simulink model "Baxter_Dyn_PID_2020"  (R2020a)
settings: Solver=FixedStepDiscrete  StartTime=0.0  StopTime=30  FixedStep=0.02  RelTol=1e-3
InitFcn:
  | initGoals
StopFcn:
  | plotSimBaxter
model workspace (MAT data in the model file):
  SL_ROS_VariableLengthArrays_MaxSizes.CommonInfo.ArrayTruncateAction = 'EmitWarning'
  SL_ROS_VariableLengthArrays_MaxSizes.MsgTypeMap = containers.Map
  SL_ROS_VariableLengthArrays_MaxSizes.MsgTypeMap.serialization.keys = {'baxter_core_msgs/JointCommand', 'sensor_msgs/JointState'}
  SL_ROS_VariableLengthArrays_MaxSizes.MsgTypeMap.serialization.values{1}(1).PropertyName = 'Command'
  SL_ROS_VariableLengthArrays_MaxSizes.MsgTypeMap.serialization.values{1}(1).DataType = 'double'
  SL_ROS_VariableLengthArrays_MaxSizes.MsgTypeMap.serialization.values{1}(1).MaxLength = 128
  SL_ROS_VariableLengthArrays_MaxSizes.MsgTypeMap.serialization.values{1}(2).PropertyName = 'Names'
  SL_ROS_VariableLengthArrays_MaxSizes.MsgTypeMap.serialization.values{1}(2).DataType = 'std_msgs/String'
  SL_ROS_VariableLengthArrays_MaxSizes.MsgTypeMap.serialization.values{1}(2).MaxLength = 19
  SL_ROS_VariableLengthArrays_MaxSizes.MsgTypeMap.serialization.values{2}(1).PropertyName = 'Effort'
  SL_ROS_VariableLengthArrays_MaxSizes.MsgTypeMap.serialization.values{2}(1).DataType = 'double'
  SL_ROS_VariableLengthArrays_MaxSizes.MsgTypeMap.serialization.values{2}(1).MaxLength = 128
  SL_ROS_VariableLengthArrays_MaxSizes.MsgTypeMap.serialization.values{2}(2).PropertyName = 'Name'
  SL_ROS_VariableLengthArrays_MaxSizes.MsgTypeMap.serialization.values{2}(2).DataType = 'std_msgs/String'
  SL_ROS_VariableLengthArrays_MaxSizes.MsgTypeMap.serialization.values{2}(2).MaxLength = 19
  SL_ROS_VariableLengthArrays_MaxSizes.MsgTypeMap.serialization.values{2}(3).PropertyName = 'Position'
  SL_ROS_VariableLengthArrays_MaxSizes.MsgTypeMap.serialization.values{2}(3).DataType = 'double'
  SL_ROS_VariableLengthArrays_MaxSizes.MsgTypeMap.serialization.values{2}(3).MaxLength = 19
  SL_ROS_VariableLengthArrays_MaxSizes.MsgTypeMap.serialization.values{2}(4).PropertyName = 'Velocity'
  SL_ROS_VariableLengthArrays_MaxSizes.MsgTypeMap.serialization.values{2}(4).DataType = 'double'
  SL_ROS_VariableLengthArrays_MaxSizes.MsgTypeMap.serialization.values{2}(4).MaxLength = 19
  SL_ROS_VariableLengthArrays_MaxSizes.MsgTypeMap.serialization.uniformity = 0
  SL_ROS_VariableLengthArrays_MaxSizes.MsgTypeMap.serialization.keyType = 'char'
  SL_ROS_VariableLengthArrays_MaxSizes.MsgTypeMap.serialization.valueType = 'any'
values from neighbouring files (symbols this model uses):
  Kp = [  1,0,0,0,0,0,0;         0,1,0,0,0,0,0;         0,0,1,0,0,0,0;         0,0,0,1,0,0,0;         0,0,0,0,1,0,0;         0,0,0,0,0,1,0;         0,0,0,0,0,0,1]    [initGoals.m]
  Kv = [  0,0,0,0,0,0,0;         0,0,0,0,0,0,0;         0,0,0,0,0,0,0;         0,0,0,0,0,0,0;         0,0,0,0,0,0,0;         0,0,0,0,0,0,0;         0,0,0,0,0,0,0]    [initGoals.m]
libraries: simulink x7, lab3lib x4
settings Model: Creator=jcollial  LastModifiedBy=spkee
settings OptimizationCC: EnhancedBackFolding=on  PassReuseOutputArgsAs=Individual arguments  ZeroExternalMemoryAtStartup=off  ZeroInternalMemoryAtStartup=off  MaxStackSize=64  OptimizeBlockOrder=speed  DifferentSizesBufferReuse=on  OptimizationCustomize=off  EfficientTunableParamExpr=on
settings DebuggingCC: ParameterTunabilityLossMsg=error
settings HardwareCC: ProdBitPerPointer=32  ProdBitPerSizeT=32  ProdBitPerPtrDiffT=32  ProdLargestAtomicFloat=None  ProdIntDivRoundTo=Undefined  ProdEndianess=Unspecified  ProdWordSize=32  ProdHWDeviceType=Generic->Unspecified (assume 32-bit Generic)  UseEmbeddedCoderFeatures=off
settings SFSimCC: MATLABDynamicMemAlloc=off
settings RTWCC: SystemTargetFile=ert.tlc  HardwareBoard=Robot Operating System (ROS)  TemplateMakefile=ert_default_tmf  Toolchain=Catkin  TargetLang=C++
settings CodeAppCC: ForceParamTrailComments=on  IgnoreCustomStorageClasses=off  OperatorAnnotations=on  SimulinkDataObjDesc=on  SFDataObjDesc=on  InsertBlockDesc=on
settings ERTTargetCC: SupportNonInlinedSFcns=on

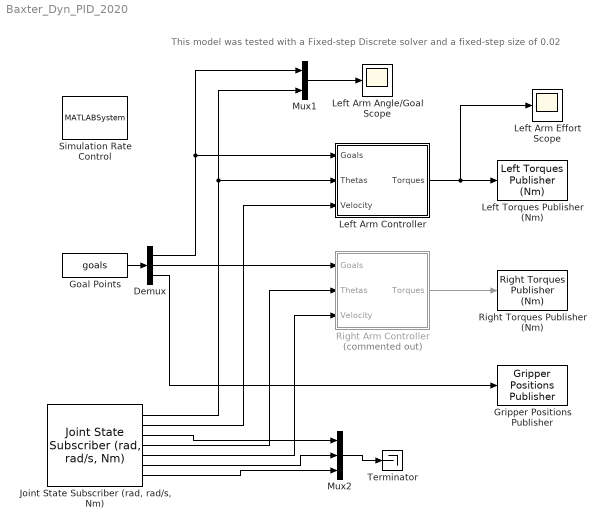
== system Baxter_Dyn_PID_2020 ==
  note: This model was tested with a Fixed-step Discrete solver and a fixed-step size of 0.02
  Demux : Demux  Outputs=3
  Goal Points : FromWorkspace  VariableName=goals  Interpolate=off  OutputAfterFinalValue=Holding final value
  Gripper Positions Publisher : lab3lib/Gripper Positions Publisher
      link override Publish: topic=/robot/end_effector/left_gripper/command  messageType=baxter_core_msgs/EndEffectorCommand
      settings: SourceProductName=Baxter
  "Joint State Subscriber (rad, rad/s, Nm)" : lab3lib/Joint State Subscriber (rad, rad//s, Nm)
      settings: SourceProductName=Baxter
  Left Arm Angle/Goal Scope : Scope
  Left Arm Controller : Subsystem
  Left Arm Effort Scope : Scope
  Left Torques Publisher (Nm) : lab3lib/Left Torques Publisher (Nm)
      settings: SourceProductName=Baxter
  Mux1 : Mux  Inputs=2
  Mux2 : Mux  Inputs=3
  Right Arm Controller : Subsystem  Commented=on
  Right Torques Publisher (Nm) : lab3lib/Right Torques Publisher (Nm)
      settings: SourceProductName=Baxter
  Simulation Rate Control : MATLABSystem  System=ExampleHelperSimulationRateControl  SampleTime=0.02
      mask Type: ExampleHelperSimulationRateControl
      mask Display: disp('Rate Control');
  Terminator : Terminator
  wires:
  Demux/1 -> Left Arm Controller/1(Goals), Mux1/1
  "Joint State Subscriber (rad, rad/s, Nm)"/1 -> Left Arm Controller/2(Thetas), Mux1/2
  Mux1/1 -> Left Arm Angle/Goal Scope/1
  Mux2/1 -> Terminator/1
  Goal Points/1 -> Demux/1
  Demux/3 -> Gripper Positions Publisher/1
  Left Arm Controller/1(Torques) -> Left Torques Publisher (Nm)/1, Left Arm Effort Scope/1
  "Joint State Subscriber (rad, rad/s, Nm)"/2 -> Left Arm Controller/3(Velocity)
  Demux/2 -> Right Arm Controller/1(Goals)
  Right Arm Controller/1(Torques) -> Right Torques Publisher (Nm)/1
  "Joint State Subscriber (rad, rad/s, Nm)"/4 -> Right Arm Controller/2(Thetas)
  "Joint State Subscriber (rad, rad/s, Nm)"/5 -> Right Arm Controller/3(Velocity)
  "Joint State Subscriber (rad, rad/s, Nm)"/3 -> Mux2/1
  "Joint State Subscriber (rad, rad/s, Nm)"/6 -> Mux2/2
  "Joint State Subscriber (rad, rad/s, Nm)"/7 -> Mux2/3

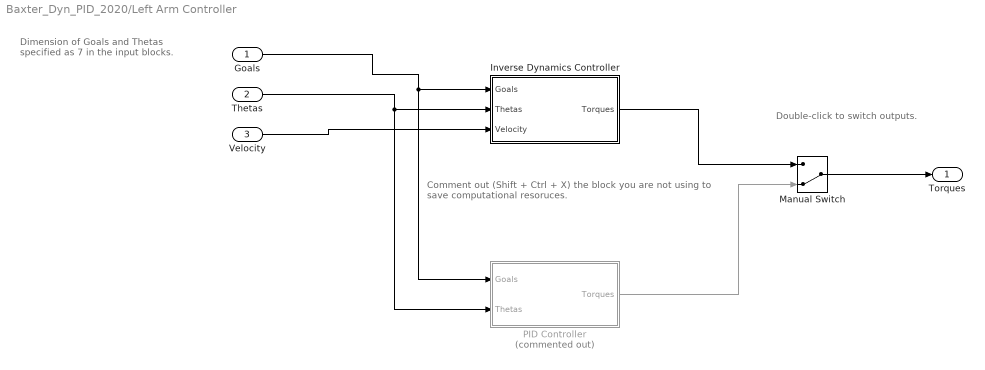
== system Baxter_Dyn_PID_2020/Left Arm Controller ==
  note: Dimension of Goals and Thetas
      | specified as 7 in the input blocks.
  note: Comment out (Shift + Ctrl + X) the block you are not using
      | to save computational resoruces.
  note: Double-click to switch outputs.
  Goals : Inport  PortDimensions=7
  Thetas : Inport  Port=2  PortDimensions=7
  Velocity : Inport  Port=3  PortDimensions=7
  Inverse Dynamics Controller : Subsystem
  Manual Switch : ManualSwitch  CurrentSetting=0
  PID Controller : Subsystem  Commented=on
  Torques : Outport
  wires:
  Goals/1 -> PID Controller/1(Goals), Inverse Dynamics Controller/1(Goals)
  Thetas/1 -> PID Controller/2(Thetas), Inverse Dynamics Controller/2(Thetas)
  Velocity/1 -> Inverse Dynamics Controller/3(Velocity)
  Manual Switch/1 -> Torques/1
  Inverse Dynamics Controller/1(Torques) -> Manual Switch/1
  PID Controller/1(Torques) -> Manual Switch/2

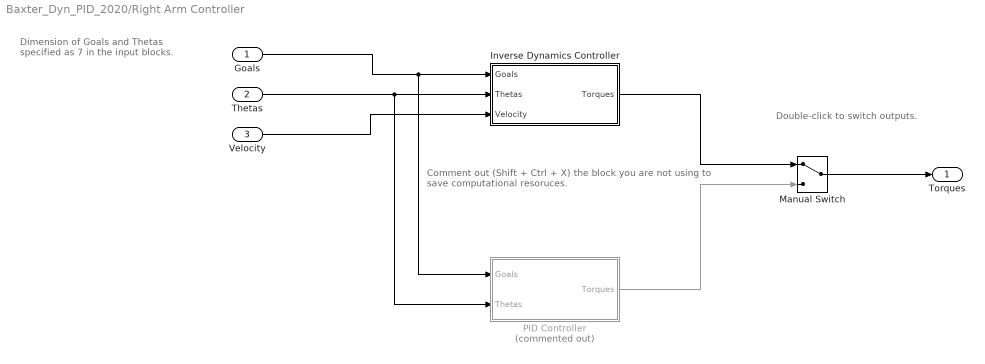
== system Baxter_Dyn_PID_2020/Right Arm Controller ==
  note: Double-click to switch outputs.
  note: Comment out (Shift + Ctrl + X) the block you are not using
      | to save computational resoruces.
  note: Dimension of Goals and Thetas
      | specified as 7 in the input blocks.
  Goals : Inport  PortDimensions=7
  Thetas : Inport  Port=2  PortDimensions=7
  Velocity : Inport  Port=3  PortDimensions=7
  Inverse Dynamics Controller : Subsystem
  Manual Switch : ManualSwitch
  PID Controller : Subsystem  Commented=on
  Torques : Outport
  wires:
  PID Controller/1(Torques) -> Manual Switch/2
  Thetas/1 -> PID Controller/2(Thetas), Inverse Dynamics Controller/2(Thetas)
  Inverse Dynamics Controller/1(Torques) -> Manual Switch/1
  Velocity/1 -> Inverse Dynamics Controller/3(Velocity)
  Goals/1 -> PID Controller/1(Goals), Inverse Dynamics Controller/1(Goals)
  Manual Switch/1 -> Torques/1

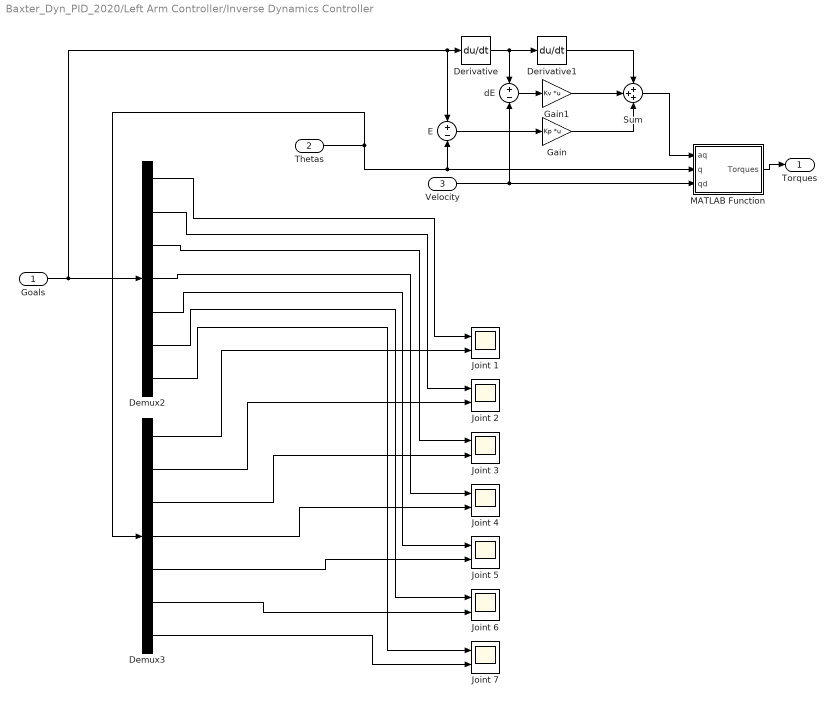
== system Baxter_Dyn_PID_2020/Left Arm Controller/Inverse Dynamics Controller ==
  Goals : Inport  PortDimensions=7
  Thetas : Inport  Port=2  PortDimensions=7
  Velocity : Inport  Port=3  PortDimensions=7
  Demux2 : Demux  Outputs=7
  Demux3 : Demux  Outputs=7
  Derivative : Derivative
  Derivative1 : Derivative
  E : Sum  Inputs=+|-
  Gain : Gain  Gain=Kp  Multiplication=Matrix(K*u)
  Gain1 : Gain  Gain=Kv  Multiplication=Matrix(K*u)
  Joint {1..7} (7 alike) : Scope  NumInputPorts=2
  MATLAB Function : MATLAB Function  TreatAsAtomicUnit=on
  Sum : Sum  Inputs=+++
  dE : Sum  Inputs=+|-
  Torques : Outport
  wires:
  MATLAB Function/1(Torques) -> Torques/1
  Demux3/3 -> Joint 3/2
  Gain/1 -> Sum/3
  Derivative1/1 -> Sum/1
  Thetas/1 -> Demux3/1, E/2, MATLAB Function/2(q)
  Derivative/1 -> Derivative1/1, dE/1
  Demux2/4 -> Joint 4/1
  Demux3/4 -> Joint 4/2
  Goals/1 -> Derivative/1, E/1, Demux2/1
  Velocity/1 -> MATLAB Function/3(qd), dE/2
  Demux3/5 -> Joint 5/2
  Demux2/1 -> Joint 1/1
  Gain1/1 -> Sum/2
  Demux3/1 -> Joint 1/2
  Demux3/7 -> Joint 7/2
  Demux3/6 -> Joint 6/2
  Demux2/3 -> Joint 3/1
  Demux2/2 -> Joint 2/1
  Demux2/6 -> Joint 6/1
  E/1 -> Gain/1
  Demux2/7 -> Joint 7/1
  Demux3/2 -> Joint 2/2
  Demux2/5 -> Joint 5/1
  dE/1 -> Gain1/1
  Sum/1 -> MATLAB Function/1(aq)

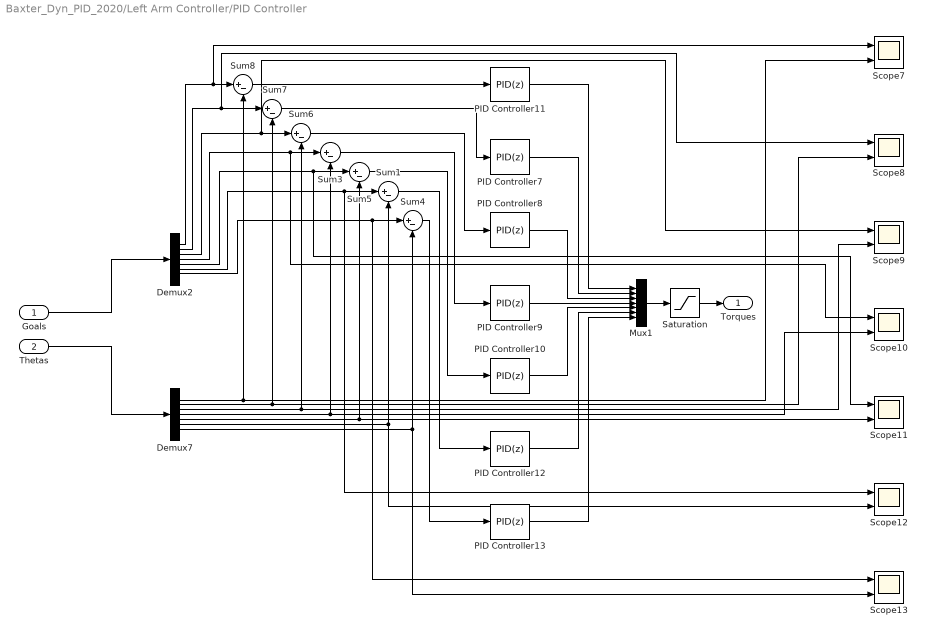
== system Baxter_Dyn_PID_2020/Left Arm Controller/PID Controller ==
  Goals : Inport  PortDimensions=7
  Thetas : Inport  Port=2  PortDimensions=7
  Demux2 : Demux  Outputs=7
  Demux7 : Demux  Outputs=7
  Mux1 : Mux  Inputs=7
  PID Controller10 : simulink/Continuous/PID Controller  Controller=PID  Form=Parallel  TimeDomain=Discrete-time  UseExternalTs=off  SampleTime=-1  IntegratorMethod=Forward Euler  FilterMethod=Forward Euler  ControllerParametersSource=internal  P=1  I=0  D=0  UseFilter=off  N=15  TunerSelectOption=Transfer Function Based (PID Tuner App)  InitialConditionSource=internal  InitialConditionForIntegrator=0  InitialConditionForFilter=0  DifferentiatorICPrevScaledInput=0  ExternalReset=none  TrackingMode=off  Kt=1  LimitOutput=off  UpperSaturationLimit=inf  LowerSaturationLimit=-inf  LinearizeAsGain=on  AntiWindupMode=none  Kb=1  POutMin=[]  POutMax=[]  IOutMin=[]  IOutMax=[]  DOutMin=[]  DOutMax=[]  NOutMin=[]  NOutMax=[]  SumOutMin=[]  SumOutMax=[]  SaturationOutMin=[]  SaturationOutMax=[]  PParamMin=[]  PParamMax=[]  IParamMin=[]  IParamMax=[]  DParamMin=[]  DParamMax=[]  NParamMin=[]  NParamMax=[]  KbParamMin=[]  KbParamMax=[]  KtParamMin=[]  KtParamMax=[]  KbOutMin=[]  KbOutMax=[]  KtOutMin=[]  KtOutMax=[]  IntegratorOutMin=[]  IntegratorOutMax=[]  FilterOutMin=[]  FilterOutMax=[]  SumI1OutMin=[]  SumI1OutMax=[]  SumI2OutMin=[]  SumI2OutMax=[]  SumI3OutMin=[]  SumI3OutMax=[]  SumI4OutMin=[]  SumI4OutMax=[]  SumDOutMin=[]  SumDOutMax=[]  DifferentiatorOutMin=[]  DifferentiatorOutMax=[]  FilterDiffOutCoefMin=[]  FilterDiffOutCoefMax=[]  ReciprocalOutMin=[]  ReciprocalOutMax=[]  SumDenOutMin=[]  SumDenOutMax=[]  SumNumOutMin=[]  SumNumOutMax=[]  DivideOutMin=[]  DivideOutMax=[]  UdiffTsProdOutMin=[]  UdiffTsProdOutMax=[]  NTsProdOutMin=[]  NTsProdOutMax=[]  UintegralTsProdOutMin=[]  UintegralTsProdOutMax=[]  UngainTsProdOutMin=[]  UngainTsProdOutMax=[]  IntegratorContinuousStateAttributes=''  IntegratorStateMustResolveToSignalObject=off  IntegratorRTWStateStorageClass=Auto  FilterContinuousStateAttributes=''  FilterStateMustResolveToSignalObject=off  FilterRTWStateStorageClass=Auto  ParallelPVariant=InternalParameters  IdealPVariant=Disabled  IVariant=InternalParameters  DVariant=InternalParameters  IntegratorVariant=Discrete  SatVariant=Disabled  AWVariant=Passthrough  PCopyVariant=Disabled  TRVariant=Disabled  FdbkBlocksVariant=Forward  IdealPFdbkVariant=Disabled  SatFdbkVariant=Disabled  DerivativeFilterVariant=Differentiator  NVariant=Passthrough  NCopyVariant=Disabled_SignalSpec  FilterICVariant=InternalICsDifferentiator  IntegratorICVariant=InternalICs  ExternalResetVariant=Disabled  TRSumVariant=Passthrough  SumFdbkVariant=Disabled  SumVariant=Sum_PID  TsampFilterVariant=InternalTs  TsampNgainVariant=Passthrough  TsampIntegralVariant=Passthrough
  PID Controller11 : simulink/Continuous/PID Controller  Controller=PID  Form=Parallel  TimeDomain=Discrete-time  UseExternalTs=off  SampleTime=-1  IntegratorMethod=Forward Euler  FilterMethod=Forward Euler  ControllerParametersSource=internal  P=16  I=0  D=8  UseFilter=on  N=15  TunerSelectOption=Transfer Function Based (PID Tuner App)  InitialConditionSource=internal  InitialConditionForIntegrator=0  InitialConditionForFilter=0  DifferentiatorICPrevScaledInput=0  ExternalReset=none  TrackingMode=off  Kt=1  LimitOutput=off  UpperSaturationLimit=inf  LowerSaturationLimit=-inf  LinearizeAsGain=on  AntiWindupMode=none  Kb=1  POutMin=[]  POutMax=[]  IOutMin=[]  IOutMax=[]  DOutMin=[]  DOutMax=[]  NOutMin=[]  NOutMax=[]  SumOutMin=[]  SumOutMax=[]  SaturationOutMin=[]  SaturationOutMax=[]  PParamMin=[]  PParamMax=[]  IParamMin=[]  IParamMax=[]  DParamMin=[]  DParamMax=[]  NParamMin=[]  NParamMax=[]  KbParamMin=[]  KbParamMax=[]  KtParamMin=[]  KtParamMax=[]  KbOutMin=[]  KbOutMax=[]  KtOutMin=[]  KtOutMax=[]  IntegratorOutMin=[]  IntegratorOutMax=[]  FilterOutMin=[]  FilterOutMax=[]  SumI1OutMin=[]  SumI1OutMax=[]  SumI2OutMin=[]  SumI2OutMax=[]  SumI3OutMin=[]  SumI3OutMax=[]  SumI4OutMin=[]  SumI4OutMax=[]  SumDOutMin=[]  SumDOutMax=[]  DifferentiatorOutMin=[]  DifferentiatorOutMax=[]  FilterDiffOutCoefMin=[]  FilterDiffOutCoefMax=[]  ReciprocalOutMin=[]  ReciprocalOutMax=[]  SumDenOutMin=[]  SumDenOutMax=[]  SumNumOutMin=[]  SumNumOutMax=[]  DivideOutMin=[]  DivideOutMax=[]  UdiffTsProdOutMin=[]  UdiffTsProdOutMax=[]  NTsProdOutMin=[]  NTsProdOutMax=[]  UintegralTsProdOutMin=[]  UintegralTsProdOutMax=[]  UngainTsProdOutMin=[]  UngainTsProdOutMax=[]  IntegratorContinuousStateAttributes=''  IntegratorStateMustResolveToSignalObject=off  IntegratorRTWStateStorageClass=Auto  FilterContinuousStateAttributes=''  FilterStateMustResolveToSignalObject=off  FilterRTWStateStorageClass=Auto  ParallelPVariant=InternalParameters  IdealPVariant=Disabled  IVariant=InternalParameters  DVariant=InternalParameters  IntegratorVariant=Discrete  SatVariant=Disabled  AWVariant=Passthrough  PCopyVariant=Disabled  TRVariant=Disabled  FdbkBlocksVariant=Forward  IdealPFdbkVariant=Disabled  SatFdbkVariant=Disabled  DerivativeFilterVariant=ForwardEulerFilter  NVariant=InternalParameters  NCopyVariant=Disabled  FilterICVariant=InternalICsFilter  IntegratorICVariant=InternalICs  ExternalResetVariant=Disabled  TRSumVariant=Passthrough  SumFdbkVariant=Disabled  SumVariant=Sum_PID  TsampFilterVariant=InternalTs  TsampNgainVariant=Passthrough  TsampIntegralVariant=Passthrough
  PID Controller12 : simulink/Continuous/PID Controller  Controller=PID  Form=Parallel  TimeDomain=Discrete-time  UseExternalTs=off  SampleTime=-1  IntegratorMethod=Forward Euler  FilterMethod=Forward Euler  ControllerParametersSource=internal  P=4  I=0  D=0  UseFilter=on  N=15  TunerSelectOption=Transfer Function Based (PID Tuner App)  InitialConditionSource=internal  InitialConditionForIntegrator=0  InitialConditionForFilter=0  DifferentiatorICPrevScaledInput=0  ExternalReset=none  TrackingMode=off  Kt=1  LimitOutput=off  UpperSaturationLimit=inf  LowerSaturationLimit=-inf  LinearizeAsGain=on  AntiWindupMode=none  Kb=1  POutMin=[]  POutMax=[]  IOutMin=[]  IOutMax=[]  DOutMin=[]  DOutMax=[]  NOutMin=[]  NOutMax=[]  SumOutMin=[]  SumOutMax=[]  SaturationOutMin=[]  SaturationOutMax=[]  PParamMin=[]  PParamMax=[]  IParamMin=[]  IParamMax=[]  DParamMin=[]  DParamMax=[]  NParamMin=[]  NParamMax=[]  KbParamMin=[]  KbParamMax=[]  KtParamMin=[]  KtParamMax=[]  KbOutMin=[]  KbOutMax=[]  KtOutMin=[]  KtOutMax=[]  IntegratorOutMin=[]  IntegratorOutMax=[]  FilterOutMin=[]  FilterOutMax=[]  SumI1OutMin=[]  SumI1OutMax=[]  SumI2OutMin=[]  SumI2OutMax=[]  SumI3OutMin=[]  SumI3OutMax=[]  SumI4OutMin=[]  SumI4OutMax=[]  SumDOutMin=[]  SumDOutMax=[]  DifferentiatorOutMin=[]  DifferentiatorOutMax=[]  FilterDiffOutCoefMin=[]  FilterDiffOutCoefMax=[]  ReciprocalOutMin=[]  ReciprocalOutMax=[]  SumDenOutMin=[]  SumDenOutMax=[]  SumNumOutMin=[]  SumNumOutMax=[]  DivideOutMin=[]  DivideOutMax=[]  UdiffTsProdOutMin=[]  UdiffTsProdOutMax=[]  NTsProdOutMin=[]  NTsProdOutMax=[]  UintegralTsProdOutMin=[]  UintegralTsProdOutMax=[]  UngainTsProdOutMin=[]  UngainTsProdOutMax=[]  IntegratorContinuousStateAttributes=''  IntegratorStateMustResolveToSignalObject=off  IntegratorRTWStateStorageClass=Auto  FilterContinuousStateAttributes=''  FilterStateMustResolveToSignalObject=off  FilterRTWStateStorageClass=Auto  ParallelPVariant=InternalParameters  IdealPVariant=Disabled  IVariant=InternalParameters  DVariant=InternalParameters  IntegratorVariant=Discrete  SatVariant=Disabled  AWVariant=Passthrough  PCopyVariant=Disabled  TRVariant=Disabled  FdbkBlocksVariant=Forward  IdealPFdbkVariant=Disabled  SatFdbkVariant=Disabled  DerivativeFilterVariant=ForwardEulerFilter  NVariant=InternalParameters  NCopyVariant=Disabled  FilterICVariant=InternalICsFilter  IntegratorICVariant=InternalICs  ExternalResetVariant=Disabled  TRSumVariant=Passthrough  SumFdbkVariant=Disabled  SumVariant=Sum_PID  TsampFilterVariant=InternalTs  TsampNgainVariant=Passthrough  TsampIntegralVariant=Passthrough
  PID Controller{7..9,13} (4 alike) : simulink/Continuous/PID Controller  Controller=PID  Form=Parallel  TimeDomain=Discrete-time  UseExternalTs=off  SampleTime=-1  IntegratorMethod=Forward Euler  FilterMethod=Forward Euler  ControllerParametersSource=internal  P=1  I=0  D=0  UseFilter=on  N=15  TunerSelectOption=Transfer Function Based (PID Tuner App)  InitialConditionSource=internal  InitialConditionForIntegrator=0  InitialConditionForFilter=0  DifferentiatorICPrevScaledInput=0  ExternalReset=none  TrackingMode=off  Kt=1  LimitOutput=off  UpperSaturationLimit=inf  LowerSaturationLimit=-inf  LinearizeAsGain=on  AntiWindupMode=none  Kb=1  POutMin=[]  POutMax=[]  IOutMin=[]  IOutMax=[]  DOutMin=[]  DOutMax=[]  NOutMin=[]  NOutMax=[]  SumOutMin=[]  SumOutMax=[]  SaturationOutMin=[]  SaturationOutMax=[]  PParamMin=[]  PParamMax=[]  IParamMin=[]  IParamMax=[]  DParamMin=[]  DParamMax=[]  NParamMin=[]  NParamMax=[]  KbParamMin=[]  KbParamMax=[]  KtParamMin=[]  KtParamMax=[]  KbOutMin=[]  KbOutMax=[]  KtOutMin=[]  KtOutMax=[]  IntegratorOutMin=[]  IntegratorOutMax=[]  FilterOutMin=[]  FilterOutMax=[]  SumI1OutMin=[]  SumI1OutMax=[]  SumI2OutMin=[]  SumI2OutMax=[]  SumI3OutMin=[]  SumI3OutMax=[]  SumI4OutMin=[]  SumI4OutMax=[]  SumDOutMin=[]  SumDOutMax=[]  DifferentiatorOutMin=[]  DifferentiatorOutMax=[]  FilterDiffOutCoefMin=[]  FilterDiffOutCoefMax=[]  ReciprocalOutMin=[]  ReciprocalOutMax=[]  SumDenOutMin=[]  SumDenOutMax=[]  SumNumOutMin=[]  SumNumOutMax=[]  DivideOutMin=[]  DivideOutMax=[]  UdiffTsProdOutMin=[]  UdiffTsProdOutMax=[]  NTsProdOutMin=[]  NTsProdOutMax=[]  UintegralTsProdOutMin=[]  UintegralTsProdOutMax=[]  UngainTsProdOutMin=[]  UngainTsProdOutMax=[]  IntegratorContinuousStateAttributes=''  IntegratorStateMustResolveToSignalObject=off  IntegratorRTWStateStorageClass=Auto  FilterContinuousStateAttributes=''  FilterStateMustResolveToSignalObject=off  FilterRTWStateStorageClass=Auto  ParallelPVariant=InternalParameters  IdealPVariant=Disabled  IVariant=InternalParameters  DVariant=InternalParameters  IntegratorVariant=Discrete  SatVariant=Disabled  AWVariant=Passthrough  PCopyVariant=Disabled  TRVariant=Disabled  FdbkBlocksVariant=Forward  IdealPFdbkVariant=Disabled  SatFdbkVariant=Disabled  DerivativeFilterVariant=ForwardEulerFilter  NVariant=InternalParameters  NCopyVariant=Disabled  FilterICVariant=InternalICsFilter  IntegratorICVariant=InternalICs  ExternalResetVariant=Disabled  TRSumVariant=Passthrough  SumFdbkVariant=Disabled  SumVariant=Sum_PID  TsampFilterVariant=InternalTs  TsampNgainVariant=Passthrough  TsampIntegralVariant=Passthrough
  Saturation : Saturate  UpperLimit=5  LowerLimit=-5
  Scope{7..13} (7 alike) : Scope  NumInputPorts=2
  Sum{1,3..8} (7 alike) : Sum  Inputs=|+-
  Torques : Outport
  wires:
  Demux7/3 -> Scope9/2, Sum6/2
  Sum8/1 -> PID Controller11/1
  Demux7/6 -> Scope12/2, Sum1/2
  Demux2/1 -> Scope7/1, Sum8/1
  Sum6/1 -> PID Controller8/1
  Sum7/1 -> PID Controller7/1
  Demux7/5 -> Scope11/2, Sum5/2
  PID Controller9/1 -> Mux1/4
  Goals/1 -> Demux2/1
  Demux2/7 -> Scope13/1, Sum4/1
  PID Controller8/1 -> Mux1/3
  Sum1/1 -> PID Controller12/1
  Saturation/1 -> Torques/1
  PID Controller10/1 -> Mux1/5
  Mux1/1 -> Saturation/1
  PID Controller7/1 -> Mux1/2
  Demux2/3 -> Scope9/1, Sum6/1
  PID Controller11/1 -> Mux1/1
  PID Controller13/1 -> Mux1/7
  Sum3/1 -> PID Controller9/1
  Demux7/7 -> Scope13/2, Sum4/2
  Demux7/2 -> Scope8/2, Sum7/2
  Demux2/6 -> Scope12/1, Sum1/1
  Demux2/5 -> Scope11/1, Sum5/1
  Sum5/1 -> PID Controller10/1
  Demux7/4 -> Scope10/2, Sum3/2
  Sum4/1 -> PID Controller13/1
  PID Controller12/1 -> Mux1/6
  Demux2/2 -> Scope8/1, Sum7/1
  Thetas/1 -> Demux7/1
  Demux2/4 -> Scope10/1, Sum3/1
  Demux7/1 -> Sum8/2, Scope7/2

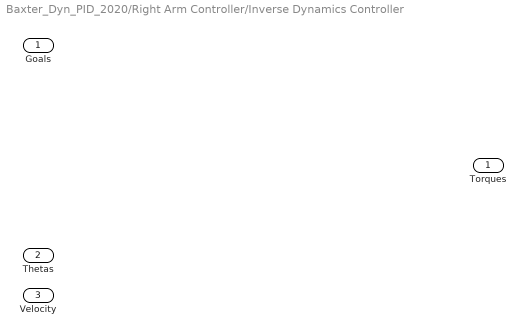
== system Baxter_Dyn_PID_2020/Right Arm Controller/Inverse Dynamics Controller ==
  Goals : Inport  PortDimensions=7
  Thetas : Inport  Port=2  PortDimensions=7
  Velocity : Inport  Port=3  PortDimensions=7
  Torques : Outport

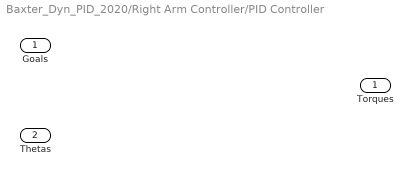
== system Baxter_Dyn_PID_2020/Right Arm Controller/PID Controller ==
  Goals : Inport  PortDimensions=7
  Thetas : Inport  Port=2  PortDimensions=7
  Torques : Outport

== matlab function Baxter_Dyn_PID_2020/Left Arm Controller/Inverse Dynamics Controller/MATLAB Function ==
  data: aq input; q input; Torques output; qd input
function Torques  = baxterdyn(aq,q,qd)
% Baxter's dynamics computed using Newton-Euler-Lagrange method.
% Author: Jose Guillermo Colli Alfaro
% Course: ECE9053A
aq
qd
q
 
% Define the constants
n=7;
%pi = sym('pi'); % Create a symbolic number that avoid the floating-point approximations inherent in the values of pi

% Mass in kg
M = [5.7004, 3.2270, 4.3127, 2.0721, 2.2467, 1.6098, 0.3509];

% Baxter lengths in meters
l1 = 0.27035;
l2 = 0.069;
l3 = 0.36435;
l4 = 0.069;
l5 = 0.37429;
l6 = 0.010;
l7 = 0.229525;

% Baxter length from joint to joint in meters
j1 = l1;
j2 = l2;
j3 = 0.102;
j4 = 0.26242;
j5 = l4;
j6 = 0.10359;
j7 = 0.2707;
j8 = l6;
j9 = 0.115975;
j10 = 0.11355;

% Gravity
g = 9.81; %m/s
 
%Assign Inputs
a = [l2, 0, l4, 0, l6, 0, 0];
d = [l1, 0, l3, 0, l5, 0, l7];
alpha = [-pi/2, pi/2, -pi/2, pi/2, -pi/2, pi/2, 0];
qdd = [aq(1),aq(2),aq(3),aq(4),aq(5),aq(6),aq(7)];
% q(2) = q(2)+pi/2;

% Define the dynamics
% Inertia
% Create an Inertia multiarray (1 for each joint)
I = zeros(3,3,n);

I(:,:,1) = [0.04709102262, 0.00012787556, 0.00614870039
            0.00012787556, 0.03766976455, 0.00078086899
            0.00614870039, 0.00078086899, 0.03595988478];
        
I(:,:,2) = [0.01175209419, -0.00030096398, 0.00207675762
           -0.00030096398,  0.0278859752, -0.00018821993
            0.00207675762, -0.00018821993, 0.02078749298];

I(:,:,3) = [0.02661733557, 0.00029270634, 0.00392189887
            0.00029270634, 0.02844355207, 0.00108389330
            0.00392189887, 0.00108389330, 0.01248008322];
        
I(:,:,4) = [0.00711582686, 0.00036036173,  0.0007459496
            0.00036036173, 0.01318227876, -0.00019663418
            0.0007459496, -0.00019663418,  0.00926852064]; 

I(:,:,5) = [0.01667742825,  0.00018403705,  0.00018657629
            0.00018403705,  0.01675457264, -0.00064732352
            0.00018657629, -0.00064732352,  0.0037463115];
        
I(:,:,6) = [ 0.00387607152, -0.00044384784, -0.00021115038
            -0.00044384784,  0.00700537914,  0.00015348067
            -0.00021115038,  0.00015348067,  0.0055275524];
        
I(:,:,7) = [ 0.00025289155,  0.00000575311, -0.00000159345
             0.00000575311,  0.0002688601,  -0.00000519818
            -0.00000159345, -0.00000519818,  0.0003074118];

% Baxter's CoM relative to the joint i
CoMS0 = [0.0178; 0.00086; 0.1913];
CoMS1 = [0.0685; 0.0027; -0.0053];
CoME0 = [-0.0028; 0.0013; 0.1809];
CoME1 = [0.0261; 0.0016; -0.0112];
CoMW0 = [-0.0017; 0.0046; 0.1395];
CoMW1 = [0.0604; 0.0070; 0.0060];
CoMW2 = [0.0020; 0.0013; 0.0186];
        
% Create Center of Mass vector of each joint relative to Oi-1. Units are in meters
% r(i-1,ci)
rc = zeros(3,n);
rc(:,1) = [0.0178; 0.00086; 0.1913]; % CoM Vector of S0
rc(:,2) = [0.0685; 0.0027; -0.0053]; % CoM Vector of S1
rc(:,3) = [-0.0028; 0.0013; 0.1809]; % CoM Vector of E0
rc(:,4) = [0.0261; 0.0016; -0.0112]; % CoM Vector of E1
rc(:,5) = [-0.0017; 0.0046; 0.1395]; % CoM Vector of W0
rc(:,6) = [0.0604; 0.0070; 0.0060];  % CoM Vector of W1
rc(:,7) = [0.0020; 0.0013; 0.0186];  % CoM Vector of W2

% Create Distance vector from origins for each joint. Units are in meters
% r(i-i,i)
r = zeros(3,n);
r(:,1) = [j2; 0; j1];   % r Vector from OS0 to OS1
r(:,2) = [j3; 0; 0];    % r Vector from OS1 to OE1
r(:,3) = [j5; 0; j4];   % r Vector from OE0 to OE1
r(:,4) = [j6; 0; 0];    % r Vector from OE1 to OW1
r(:,5) = [j8; 0; j7];   % r Vector from OW0 to OW1
r(:,6) = [j9; 0; 0];    % r Vector from OW1 to OW2
r(:,7) = [0; 0; j10];   % r Vector from OW2 to h

 
% Create Distance vector from origins of next joint to CoM. Units are in meters
% r(i,ci)
brc = zeros(3,n);
brc(:,1) = -(r(:,1)-rc(:,1));   % rc Vector from OS1 to CoM_S0
brc(:,2) = -(r(:,2)-rc(:,2));   % rc Vector from OE1 to CoM_S1
brc(:,3) = -(r(:,3)-rc(:,3));   % rc Vector from OE1 to CoM_E0
brc(:,4) = -(r(:,4)-rc(:,4));   % rc Vector from OW1 to CoM_E1
brc(:,5) = -(r(:,5)-rc(:,5));   % rc Vector from OW1 to CoM_W0
brc(:,6) = -(r(:,6)-rc(:,6));   % rc Vector from h to CoM_W1
brc(:,7) = -(r(:,7)-rc(:,7));   % rc Vector from h to CoM_W2


% Homogeneous Transformation Matrices
T01 = [cos(q(1)),   0,              sin(q(1))*sin(alpha(1)),    a(1)*cos(q(1));
       sin(q(1)),   0,             -cos(q(1))*sin(alpha(1)),    a(1)*sin(q(1));
       0,           sin(alpha(1)),  0,                          d(1);
       0,           0,              0,                          1];

T12 = [cos(q(2)),   0,              sin(q(2))*sin(alpha(2)),    0;
       sin(q(2)),   0,             -cos(q(2))*sin(alpha(2)),    0;
       0,           sin(alpha(2)),  0,                          0;
       0,           0,              0,                          1];
   
T23 = [cos(q(3)),   0,              sin(q(3))*sin(alpha(3)),    a(3)*cos(q(3));
       sin(q(3)),   0,             -cos(q(3))*sin(alpha(3)),    a(3)*sin(q(3));
       0,           sin(alpha(3)),  0,                          d(3);
       0,           0,              0,                          1];
   
T34 = [cos(q(4)),   0,              sin(q(4))*sin(alpha(4)),    0;
       sin(q(4)),   0,             -cos(q(4))*sin(alpha(4)),    0;
       0,           sin(alpha(4)),  0,                          0;
       0,           0,              0,                          1];
   
T45 = [cos(q(5)),   0,              sin(q(5))*sin(alpha(5)),    a(5)*cos(q(5));
       sin(q(5)),   0,             -cos(q(5))*sin(alpha(5)),    a(5)*sin(q(5));
       0,           sin(alpha(5)),  0,                          d(5);
       0,           0,              0,                          1];
   
T56 = [cos(q(6)),   0,              sin(q(6))*sin(alpha(6)),    0;
       sin(q(6)),   0,             -cos(q(6))*sin(alpha(6)),    0;
       0,           sin(alpha(6)),  0,                          0;
       0,           0,              0,                          1];
   
T67 = [cos(q(7)),  -sin(q(7))*cos(alpha(7)),    sin(q(7))*sin(alpha(7)),    0;
       sin(q(7)),   cos(q(7))*cos(alpha(7)),   -cos(q(7))*sin(alpha(7)),    0;
       0,           sin(alpha(7)),              cos(alpha(7)),              d(7);
       0,           0,                          0,                          1];
   
% Create Transformation Matrices for each joint 
T02 = (T01*T12);
T03 = (T02*T23);
T04 = (T03*T34);
T05 = (T04*T45);
T06 = (T05*T56);
T07 = (T06*T67);


% Rotation Matrices
R01 = T01((1:3),(1:3));
R12 = T12((1:3),(1:3));
R23 = T23((1:3),(1:3));
R34 = T34((1:3),(1:3));
R45 = T45((1:3),(1:3));
R56 = T56((1:3),(1:3));
R67 = T67((1:3),(1:3));

R78 = eye(3,3); % Joint doesn't exist

R02 = T02((1:3),(1:3));
R03 = T03((1:3),(1:3));
R04 = T04((1:3),(1:3));
R05 = T05((1:3),(1:3));
R06 = T06((1:3),(1:3));
R07 = T07((1:3),(1:3));

RBase = {R01 R02 R03 R04 R05 R06 R07};
RJoint = {R01 R12 R23 R34 R45 R56 R67 R78};

% z axis wrt frame 0
z = zeros(3,(n+1));
z(:,1) = [0; 0; 1];     %Zn-1
z(:,2) = T01((1:3),3);  %Zn-1
z(:,3) = T02((1:3),3);  %Zn-1
z(:,4) = T03((1:3),3);  %Zn-1
z(:,5) = T04((1:3),3);  %Zn-1
z(:,6) = T05((1:3),3);  %Zn-1
z(:,7) = T06((1:3),3);  %Zn-1
z(:,8) = T07((1:3),3);

% Outward Iteration
ac = zeros(3,(n+1));
omega = zeros(3,(n+1));
al = zeros(3,(n+1)); % alpha
ae = zeros(3,(n+1));

% Initial conditions
ae(:,1) = [0; 0; g];

% In this case, because matlab index starts in 1, the previous joint is i
% and current joint is i+1
for i = 1:n
    omega(:,i+1) = RJoint{i}'*omega(:,i) + RBase{i}'*z(:,i)*qd(i);
    al(:,i+1) = RJoint{i}'*al(:,i) + RBase{i}'*z(:,i)*qdd(i) + cross(omega(:,i+1),(RBase{i}'*z(:,i)*qd(i)));
    ae(:,i+1) = RJoint{i}'*ae(:,i) + cross(al(:,i+1),r(:,i)) + cross(omega(:,i+1),cross(omega(:,i+1),r(:,i)));
    ac(:,i+1) = RJoint{i}'*ae(:,i) + cross(al(:,i+1),brc(:,i)) + cross(omega(:,i+1),cross(omega(:,i+1),brc(:,i)));
end


% Inward Iterations
% Terminal conditions
f = zeros(3,(n+1));
tau = zeros(3,(n+1));
% ATau = zeros(n,1);
Torques = zeros(n,1);

% ac(i+1), al(i+1), omega(i+1) refers to ac(current joint), al(current joint), omega(current joint)
for i = n:-1:1
    f(:,i) = RJoint{i+1}*f(:,(i+1)) + M(i)*ac(:,(i+1)); 
    tau(:,i) = RJoint{i+1}*tau(:,i+1) - cross(f(:,i),rc(:,i)) + cross((RJoint{i+1}*f(:,(i+1))),brc(:,i)) + I(:,:,n)*al(:,(i+1)) + cross(omega(:,(i+1)),(I(:,:,n)*omega(:,(i+1))));
    %ATau(:,i) = tau(:,i)'*RJoint{i}'*z(:,1);
    Torques(i) = tau(:,i)'*RJoint{i}'*z(:,1)
end
